simulink subsystem "xrelsens"  (R2022b)
settings: Solver=VariableStepAuto  StartTime=0.0  StopTime=10.0  RelTol=1e-3
libraries: nesl_utility x9, sm_lib x1
settings Model: Creator=abhij  LastModifiedBy=abhij

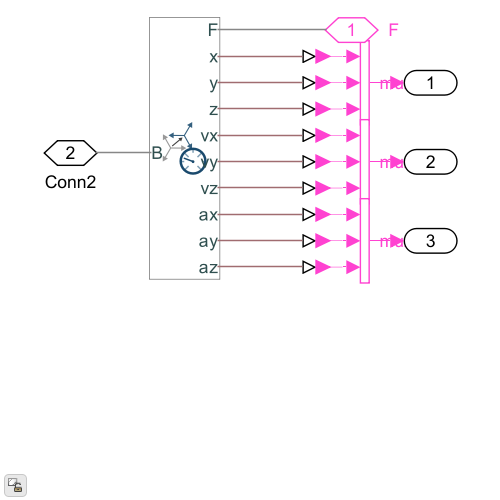
[thumbnail: Simulink's stored preview of the top-level diagram]
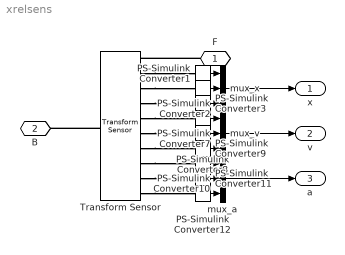
== system xrelsens ==
  PS-Simulink Converter{1..3,7..12} (9 alike) : nesl_utility/PS-Simulink Converter  PhysicalDomain=network_engine_domain  SubClassName=ps_output  LeftPortType=input  RightPortType=output  PseudoPeriodic=off  Frequencies=[]  VectorFormat=inherit  Unit=inherit  AffineConversion=off
  Transform Sensor : sm_lib/Frames and Transforms/Transform Sensor  MeasurementFrame=Base  SenseAngle=off  SenseAxis=off  SenseQ=off  SenseR=off  SenseRotationSequence=off  RotationSequence=XYX  SenseOmegaX=off  SenseOmegaY=off  SenseOmegaZ=off  SenseQDot=off  SenseRDot=off  SenseAlphaX=off  SenseAlphaY=off  SenseAlphaZ=off  SenseQDDot=off  SenseRDDot=off  SenseX=on  SenseY=on  SenseZ=on  SenseRad=off  SenseAzim=off  SenseDist=off  SenseInc=off  SenseXDot=on  SenseYDot=on  SenseZDot=on  SenseRadDot=off  SenseAzimDot=off  SenseDistDot=off  SenseIncDot=off  SenseXDDot=on  SenseYDDot=on  SenseZDDot=on  SenseRadDDot=off  SenseAzimDDot=off  SenseDistDDot=off  SenseIncDDot=off
  mux_a : Mux  Inputs=3
  mux_v : Mux  Inputs=3
  mux_x : Mux  Inputs=3
  F : PMIOPort  Side=Left
  B : PMIOPort  Port=2  Side=Left
  x : Outport
  v : Outport  Port=2
  a : Outport  Port=3
  wires:
  PS-Simulink Converter1/1 -> mux_x/1
  PS-Simulink Converter2/1 -> mux_x/2
  PS-Simulink Converter9/1 -> mux_v/3
  PS-Simulink Converter8/1 -> mux_v/2
  PS-Simulink Converter10/1 -> mux_a/1
  PS-Simulink Converter11/1 -> mux_a/2
  PS-Simulink Converter12/1 -> mux_a/3
  mux_x/1 -> x/1
  PS-Simulink Converter3/1 -> mux_x/3
  PS-Simulink Converter7/1 -> mux_v/1
  mux_a/1 -> a/1
  mux_v/1 -> v/1
  connections:
  Transform Sensor/RConn3 -- PS-Simulink Converter2/LConn1
  Transform Sensor/RConn8 -- PS-Simulink Converter10/LConn1
  Transform Sensor/RConn2 -- PS-Simulink Converter1/LConn1
  Transform Sensor/RConn4 -- PS-Simulink Converter3/LConn1
  Transform Sensor/RConn10 -- PS-Simulink Converter12/LConn1
  Transform Sensor/RConn7 -- PS-Simulink Converter9/LConn1
  Transform Sensor/RConn6 -- PS-Simulink Converter8/LConn1
  Transform Sensor/RConn5 -- PS-Simulink Converter7/LConn1
  Transform Sensor/RConn9 -- PS-Simulink Converter11/LConn1
  F/RConn1 -- Transform Sensor/RConn1
  Transform Sensor/LConn1 -- B/RConn1
